simulink model "Lab_4"  (R2022b)
settings: Solver=VariableStepAuto  StartTime=0.0  StopTime=30  RelTol=1e-3
settings Model: Creator=am331  LastModifiedBy=am331

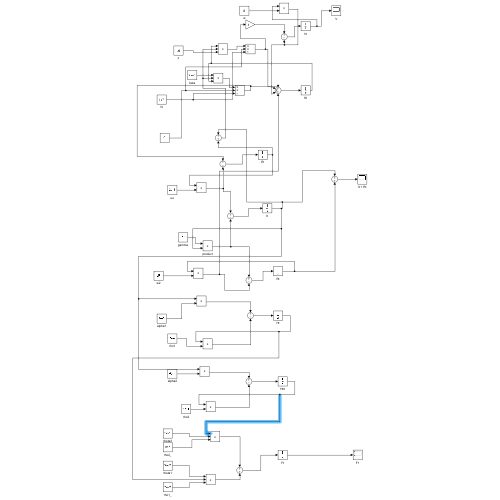
[thumbnail: Simulink's stored preview of the top-level diagram]
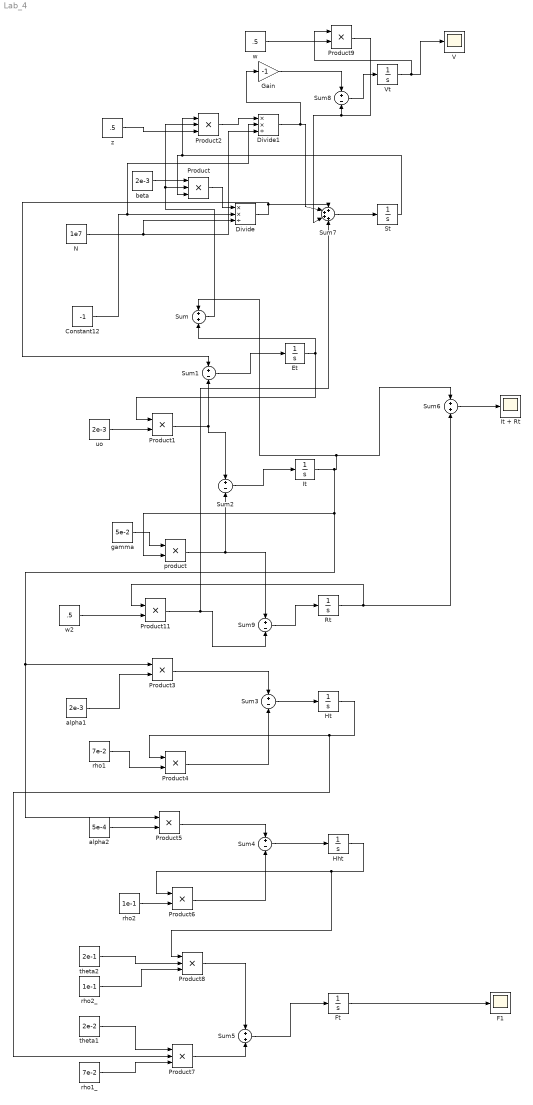
== system Lab_4 ==
  Constant12 : Constant  Value=-1
  Divide : Product  Inputs=**/
  Divide1 : Product  Inputs=**/
  Et : Integrator  InitialCondition=6e5
  F1 : Scope
  Ft : Integrator  InitialCondition=6.5e3
  Gain : Gain  Gain=-1
  Hht : Integrator  InitialCondition=188
  Ht : Integrator  InitialCondition=7e2
  It : Integrator  InitialCondition=3e4
  It + Rt : Scope
  N : Constant  Value=1e7
  Product{,2,7..8} (4 alike) : Product  Inputs=3
  Product{1,3..6,9,11} (7 alike) : Product
  Rt : Integrator  InitialCondition=2.3e5
  St : Integrator  InitialCondition=9e6
  Sum : Sum
  Sum{1..4,8..9} (6 alike) : Sum  Inputs=+-
  Sum5 : Sum
  Sum6 : Sum
  Sum7 : Sum  Inputs=++++
  V : Scope
  Vt : Integrator  InitialCondition=9e6
  alpha1 : Constant  Value=2e-3
  alpha2 : Constant  Value=5e-4
  beta : Constant  Value=2e-3
  gamma : Constant  Value=5e-2
  product : Product
  rho1 : Constant  Value=7e-2
  rho1_ : Constant  Value=7e-2
  rho2 : Constant  Value=1e-1
  rho2_ : Constant  Value=1e-1
  theta1 : Constant  Value=2e-2
  theta2 : Constant  Value=2e-1
  uo : Constant  Value=2e-3
  w : Constant  Value=.5
  w2 : Constant  Value=.5
  z : Constant  Value=.5
  wires:
  Divide/1 -> Sum7/1, Sum1/1
  N/1 -> Divide1/3, Divide/3
  beta/1 -> Product/1
  St/1 -> Product2/1, Product/3
  Et/1 -> Product1/1, Sum/2
  It/1 -> Product3/1, Product5/1, product/2, Sum6/1, Sum/1
  Sum/1 -> Product2/2, Product/2
  Product/1 -> Divide/1
  Product1/1 -> Sum2/1, Sum1/2
  Sum1/1 -> Et/1
  gamma/1 -> product/1
  product/1 -> Sum9/1, Sum2/2
  Sum2/1 -> It/1
  Sum3/1 -> Ht/1
  Product3/1 -> Sum3/1
  Ht/1 -> Product7/2, Product4/1
  Product4/1 -> Sum3/2
  Product5/1 -> Sum4/1
  Hht/1 -> Product8/1, Product6/1
  rho2/1 -> Product6/2
  Product6/1 -> Sum4/2
  Sum4/1 -> Hht/1
  Product7/1 -> Sum5/2
  Product8/1 -> Sum5/1
  Sum5/1 -> Ft/1
  Sum6/1 -> It + Rt/1
  Ft/1 -> F1/1
  Constant12/1 -> Divide1/2, Divide/2
  uo/1 -> Product1/2
  alpha1/1 -> Product3/2
  rho1/1 -> Product4/2
  alpha2/1 -> Product5/2
  theta2/1 -> Product8/2
  rho2_/1 -> Product8/3
  theta1/1 -> Product7/1
  rho1_/1 -> Product7/3
  z/1 -> Product2/3
  Sum7/1 -> St/1
  Product2/1 -> Divide1/1
  Divide1/1 -> Gain/1, Sum7/2
  Gain/1 -> Sum8/1
  Vt/1 -> Product9/1, V/1
  Sum8/1 -> Vt/1
  w/1 -> Product9/2
  Product9/1 -> Sum7/3, Sum8/2
  Rt/1 -> Product11/1, Sum6/2
  w2/1 -> Product11/2
  Product11/1 -> Sum7/4, Sum9/2
  Sum9/1 -> Rt/1
